simulink model "LM_TOS_0107_FIX"  (R2018b)
settings: Solver=FixedStepDiscrete  StartTime=0.0  StopTime=inf  FixedStep=0.005  RelTol=1e-3
PostLoadFcn:
  | if any(exist('dsrtsu_mdlpostloadfcn', 'file') ~= 0), dsrtsu_mdlpostloadfcn('Execute', bdroot); end
libraries: rtican x35
(part 1 of 11)
settings Model: DSRTSU_INTERNAL_RTI_VER=540  DSRTSU_INTERNAL_RTI_TYPE=rti1401  RTICANMMDATA=struct('GeneralSetupData',struct('modelroot','D:\00_Work\00_ZOP\00_ZOP_Demo_sim\LaneModel_20210107_1_CYX_FixHMI','generalsettings',struct('filesettings',struct('destfolder',struct('Name','RTICANMM_FILES','Check',1),'buildfolder',struct('Name','.','Check',1),'AbsDestfolder',struct('Name','D:\00_Work\00_ZOP\00_ZOP_Demo_sim\LaneModel_20210107_1_CYX_FixHMI\RTICANMM_FILES'),'AbsBuildfolder',struct('Name','D:\00_Work\00_ZOP\00_ZOP_Demo_sim\LaneModel_20210107_1_CYX_FixHMI'))),'options',struct('addpaths',1,'rmpaths',1,'addtrcexclusion',logical(1),'cannavigator',struct('checkmonitoring',0),'show_usrtrc',0,'use_usrtrc',0),'advanced',struct('options',ones(1,100)),'MPSetup',{{}},'RTI',struct('Type','RTI1401','Ver','7.12','Date','02-May-2019'),'modelname','LM_TOS','block','LM_TOS'))  DSRTSU_INTERNAL_RTIFPGA=130  Creator=only  LastModifiedBy=only
settings OptimizationCC: BlockReduction=off  ConditionallyExecuteInputs=off  DefaultUnderspecifiedDataType=single  BufferReuse=off  EnhancedBackFolding=on  ExpressionFolding=off  PassReuseOutputArgsThreshold=0  LocalBlockOutputs=off  OptimizeBlockOrder=speed  DifferentSizesBufferReuse=on
settings DebuggingCC: ParameterTunabilityLossMsg=error
settings HardwareCC: ProdBitPerPointer=32  ProdBitPerSizeT=32  ProdBitPerPtrDiffT=32  ProdLargestAtomicInteger=Integer  ProdEndianess=BigEndian  ProdWordSize=32  ProdHWDeviceType=Custom Processor->Custom  TargetIntDivRoundTo=Zero  TargetEndianess=BigEndian  TargetHWDeviceType=Custom Processor->Custom
settings ModelReferenceCC: ModelReferenceNumInstancesAllowed=Single
settings SFSimCC: MATLABDynamicMemAlloc=off
settings RTWCC: SystemTargetFile=rti1401.tlc  MakeCommand=make_rti  TemplateMakefile=rti1401.tmf  Description=dSPACE DS1401 Hardware Platform  GenerateReport=on  LaunchReport=on
settings CodeAppCC: OperatorAnnotations=on
settings STFCustomTargetCC: ParMdlRefBuildCompliant=on  SystemTargetFile=rti1401.tlc
settings GRTTargetCC: TargetLangStandard=C89/C90 (ANSI)  CompOptLevelCompliant=off  ConcurrentExecutionCompliant=off  CombineOutputUpdateFcns=off  MatFileLogging=off  CPPClassGenCompliant=off  UseToolchainInfoCompliant=off

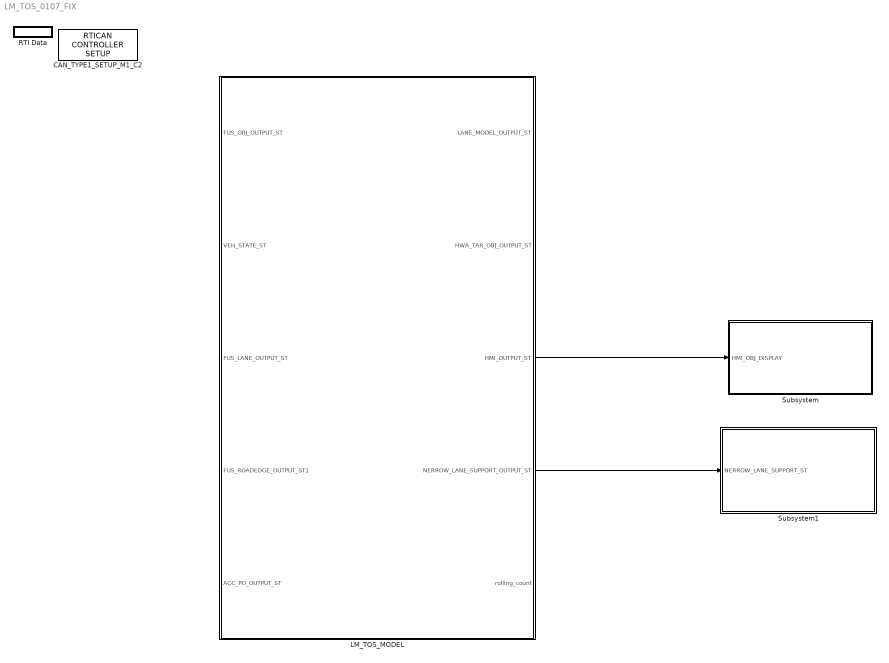
== system LM_TOS_0107_FIX ==
  CAN_TYPE1_SETUP_M1_C2 : rtican/RTICAN CONTROLLER SETUP   Reserved1=[]  Reserved2=[]  Reserved3=[]  Reserved4=[]  AcceptanceMask=[]  ArbitrationField=[]  Parameters=[]  SFcnRTICANSettings=[]  MS_Struct=[]  BoardTypeNo=[]  BoardNo=[]  ChannelNo=[]  DialogFcn=[]  UnitName=[]  Revision=[]  UnitValues=[]  DSProperties=struct('RTI',struct('Version',uint32(12),'BlockType',struct('isSLSource',uint8(0),'isSLSink',uint8(0),'isHWSource',uint8(0),'isHWSink',uint8(0),'isSetup',uint8(1),'isInline',uint8(1),'isNonInline',uint8(0),'isInterrupt',uint8(0),'isChannelwise',uint8(0)),'IOBoardType','RTICAN','UnitType','NON_MESSAGE','Identifier','MASTER','DialogType','ML','BlockSet','RTICAN','SlaveProcessor','CAN'))  RTIBlockInterface=struct('InputPortsWidth',int32(0),'InputPortsActive',0,'OutputPortsWidth',int32(0),'OutputPortsActive',0,'DialogFcn','rtican_master_setup_gui','BlockDisplay',{{['CAN CONTROLLER\n SETUP'],'center'}},'IconTransparency','on','InitLevel',3,'IWork',{{{'',uint32(2)}}},'BlockName',struct('Token',{{'CAN_TYPE','_SETUP_M','_C'}},'BlockParam',{{'BoardTypeNo','BoardNo','ChannelNo'}}),'ParameterTunableNames',{{}})  RTIBlockParameters="struct('BoardTypeNo',{{1,'OFF',[]}},'BoardNo',{{1,'ON',[1 16]}},'ChannelNo',{{2,'ON',[1 2]}},'AcceptanceMask',{{0,'OFF',[]}},'ArbitrationField',{{0,'OFF',[]}},'Parameters',{{struct('Config',struct('Baudrate',500,'SampleMode',1,'UsedParamSet',1,'validSettings',1,'isBTRvalues',0,'Advanced',struct('Baudrate',{500,500,500},'Frequency',{24000000,36000000,64000000},'Settings',{struct('SMPL',0,'BRP',0,'NBT',24,'TSEG1',15,'TSEG2',6,'SJW',3,'SP',70),struct('SMPL',0,'BRP',1,'NBT',18,'TSEG1',14,'TSEG2',1,'SJW',1,'SP',88),struct('SMPL',0,'BRP',3,'NBT',16,'TSEG1',12,'TSEG2',1,'SJW',1,'SP',87)},'BTR0',{192,65,67},'BTR1',{111,30,28})),'configType',1,'Options',struct('DataFileSelected',1,'DataFileName',{{'c:\\users\\only\\desktop\\mab_ipc_v1.8.dbc'}},'DataFileDate',{{['28-12月-2020 13:33:19']}},'InterfaceFcn','rtican_dbc_file_parser','InterfaceFcnFileName','','LabelConfigType','volatile','AcceptanceMaskSelected',0,'MsgDataType','AllwaysDouble','NumType','hex','MaskType','STD','AcceptanceMask',0,'ArbitrationField',0,'UseMultipleMessageAccess',0),'RxReceiveStdOptions',struct('RxServiceStdEnabled',0,'RxServiceStdMsgIdent',1000,'RxServiceStdIdentNumType',1,'RxServiceStdIdentMask',0,'RxServiceStdMaskNumType',1,'RxServiceStdQueueSize',64),'RxReceiveXtdOptions',struct('RxServiceXtdEnabled',0,'RxServiceXtdMsgIdent',1001,'RxServiceXtdIdentNumType',1,'RxServiceXtdIdentMask',0,'RxServiceXtdMaskNumType',1,'RxServiceXtdQueueSize',64),'PartialNetworkingOptions',struct('switchedon',0,'format',1,'idmask',['    XXXXX XXXXXXXX XXXXXXXX XXXXXXXX'],'idcode','0','idfilter','0','datamaskused',0,'datalength',1,'datamask','0x0000000000000000','partialnetworkenable',0),'general',struct('Termination_common',1,'Termination_C252',1,'BusConfigurationRegister',0,'Transceiver','ISO11898','isFromLib',0)),'OFF',[]}},'CCPParameters',{{struct('CRO',struct('Format','STD','NumFormat','hex','Id',1639),'DTO',struct('Format','STD','NumFormat','hex','Id',2017),'StationAdr',struct('NumFormat','hex','Value',57),'StationId',struct('Value',['dSPACE CCP Service']),'Enabled',0),'OFF',[]}},'XCPParameters',{{struct('MASTER',struct('Format','STD','NumFormat','hex','Id',256),'SLAVE',struct('Format','STD','NumFormat','hex','Id',510),'Enabled',0,'PIDTransmissionEnabled',0),'OFF',[]}},'GroupId',{{struct('Group',{{'RTICAN'}},'No',1,'Behavior',{{'EVER'}},'BlockType',{{'SOURCE'}},'NameChangeFlag',1),'OFF',[]}},'SFcnRTICANSettings',{{struct('Baudrate',500,'configType',1,'AdvancedConfig',struct('Frequency',{},'BTR0',{},'BTR1',{}),'UsedParamSet',1,'STDMaskSelected','no','XTDMaskSelected','no','BoardType','DS1','BoardNo',1,'ControllerNo',2,'Transceiver','ISO11898','BusConfigRegister',0,'TerminationRes',120,'UseMultipleMessageAccess','no','STDRXSrvcUsed','no','STDRXSrvcMsgId',1000,'STDRXSrvcMsgMask',0,'STDRXSrvcQueueSize',64,'XTDRXSrvcUsed','no','XTDRXSrvcMsgId',1001,'XTDRXSrvcQueueSize',64,'XTDRXSrvcMsgMask',0,'PN_IsPNTransciever',0,'PN_IsPNEnabled',0,'PN_MsgFormat',1,'PN_idcode',0,'PN_idmask',2047,'PN_datamaskused',0,'PN_datalength',0,'PN_datamask',['0xFF, 0xFF, 0xFF, 0xFF, 0xFF, 0xFF, 0xFF, 0xFF']),'OFF',[]}},'SFcnRTICCPSettings',{{struct('CRO',struct('Format','STD','NumFormat','hex','Id',1639),'DTO',struct('Format','STD','NumFormat','hex','Id',2017),'StationAdr',struct('NumFormat','hex','Value',57),'StationId',struct('Value',['dSPACE CCP Service']),'Enabled',0),'OFF',[]}},'SFcnRTIXCPSettings',{{struct('MASTER',struct('Format','STD','NumFormat','hex','Id',256),'SLAVE',struct('Format','STD','NumFormat','hex','Id',510),'Enabled',0,'PIDTransmissionEnabled',0),'OFF',[]}},'TLCFileName',{{'rtican_master_setup','OFF',[]}})"  RTISFcnParameters=struct('SFcnRTICANSettings','struct','SFcnRTICCPSettings','struct','SFcnRTIXCPSettings','struct','AcceptanceMask','int32','ArbitrationField','int32','TLCFileName','char')  RTIBlockParaDefault="struct('BoardTypeNo',4302,'BoardNo',1,'ChannelNo',1,'AcceptanceMask',0,'ArbitrationField',0,'Parameters',struct('Config',struct('Baudrate',500,'SampleMode',1,'UsedParamSet',1,'validSettings',1,'isBTRvalues',0,'Advanced',struct('Frequency',16000000,'BTR0',64,'BTR1',28,'Settings',struct('SMPL',0,'BRP',0,'NBT',16,'TSEG1',12,'TSEG2',1,'SJW',1,'SP',87))),'configType',1,'Options',struct('DataFileSelected',0,'DataFileName',{{['<no datafile support>']}},'DataFileDate',{{''}},'InterfaceFcn','rtican_dbc_file_parser','InterfaceFcnFileName','','LabelConfigType','volatile','AcceptanceMaskSelected',0,'MsgDataType','AllwaysDouble','NumType','hex','MaskType','STD','AcceptanceMask',0,'ArbitrationField',0,'UseMultipleMessageAccess',0),'RxReceiveStdOptions',struct('RxServiceStdEnabled',0,'RxServiceStdMsgIdent',1000,'RxServiceStdIdentNumType',1,'RxServiceStdIdentMask',0,'RxServiceStdMaskNumType',1,'RxServiceStdQueueSize',64),'RxReceiveXtdOptions',struct('RxServiceXtdEnabled',0,'RxServiceXtdMsgIdent',1001,'RxServiceXtdIdentNumType',1,'RxServiceXtdIdentMask',0,'RxServiceXtdMaskNumType',1,'RxServiceXtdQueueSize',64),'PartialNetworkingOptions',struct('switchedon',0,'format',1,'idmask',['    XXXXX XXXXXXXX XXXXXXXX XXXXXXXX'],'idcode','0','idfilter','0','datamaskused',0,'datalength',1,'datamask','0x0000000000000000','partialnetworkenable',0),'general',struct('Termination_common',1,'Termination_C252',1,'BusConfigurationRegister',0,'Transceiver','ISO11898','isFromLib',1)),'CCPParameters',struct('CRO',struct('Format','STD','NumFormat','hex','Id',1639),'DTO',struct('Format','STD','NumFormat','hex','Id',2017),'StationAdr',struct('NumFormat','hex','Value',57),'StationId',struct('Value',['dSPACE CCP Service']),'Enabled',0),'XCPParameters',struct('MASTER',struct('Format','STD','NumFormat','hex','Id',256),'SLAVE',struct('Format','STD','NumFormat','hex','Id',510),'Enabled',0,'PIDTransmissionEnabled',0),'GroupId',struct('Group',{{'RTICAN'}},'No',1,'Behavior',{{'EVER'}},'BlockType',{{'SOURCE'}},'NameChangeFlag',1),'SFcnRTICANSettings',struct('Baudrate',500,'configType',1,'AdvandedConfig',struct('Frequency',16000000,'BTR0','0x40','BTR1','0x1C'),'UsedParamSet',1,'STDMaskSelected','no','XTDMaskSelected','no','BoardType','DS4302','BoardNo',1,'ControllerNo',1,'Transceiver','ISO11898','BusConfigRegister',0,'TerminationRes',120,'UseMultipleMessageAccess','no','STDRXSrvcUsed','no','STDRXSrvcMsgId',1000,'STDRXSrvcMsgMask',0,'STDRXSrvcQueueSize',64,'XTDRXSrvcUsed','no','XTDRXSrvcMsgId',1001,'XTDRXSrvcQueueSize',64,'XTDRXSrvcMsgMask',0),'SFcnRTICCPSettings',struct('CRO',struct('Format','STD','NumFormat','hex','Id',1639),'DTO',struct('Format','STD','NumFormat','hex','Id',2017),'StationAdr',struct('NumFormat','hex','Value',57),'StationId',struct('Value',['dSPACE CCP Service']),'Enabled',0),'SFcnRTIXCPSettings',struct('MASTER',struct('Format','STD','NumFormat','hex','Id',256),'SLAVE',struct('Format','STD','NumFormat','hex','Id',510),'Enabled',0,'PIDTransmissionEnabled',0),'TLCFileName','rtican_master_setup')"
      settings: AttributesFormatString=Group Id: RTICAN1\n  SourceProductName=dSPACE RTI CAN Blockset
  LM_TOS_MODEL : Subsystem
  RTI Data : Subsystem  Tag=struct('RTIDataServer',struct('RTIDataServerVs','2','RTIModelDescription','struct(''main'',''LM_TOS'',''sub'','''',''isMp'',0)'))  LoadFcn="if exist('rtidc'), try,  rtidc('DataHostBlockClbLoad', gcbh); catch, disp(['Warning: ''LoadFcn'' for RTI Data block failed: ' lasterr]); end, end,"  mask(RTI_DATA_HOST){}
      mask help:
      | RTI Data Block.
      | This block is used by RTI to store internal model-dependent data.
      | Please keep this block on the root level of the model. Deleting this block will result in data loss.
      |
      | NEVER DELETE OR COPY THIS BLOCK!
      settings: CopyFcn="if exist('rtidc'), try,  rtidc('DataHostBlockClbCopy', gcbh); catch, disp(['Warning: ''CopyFcn'' for RTI Data block failed: ' lasterr]); end, end,"  DeleteFcn="if exist('rtidc'), try,  rtidc('DataHostBlockClbDelete', gcbh); catch, disp(['Warning: ''DeleteFcn'' for RTI Data block failed: ' lasterr]); end, end,"  ModelCloseFcn="if exist('rtidc'), try,  rtidc('DataHostBlockClbModelClose', gcbh); catch, disp(['Warning: ''ModelCloseFcn'' for RTI Data block failed: ' lasterr]); end, end,"  PreSaveFcn="if exist('rtidc'), try,  rtidc('DataHostBlockClbPreSave', gcbh); catch, disp(['Warning: ''PreSaveFcn'' for RTI Data block failed: ' lasterr]); end, end,"  PostSaveFcn="if exist('rtidc'), try,  rtidc('DataHostBlockClbPostSave', gcbh); catch, disp(['Warning: ''PostSaveFcn'' for RTI Data block failed: ' lasterr]); end, end,"  NameChangeFcn="if exist('rtidc'), try,  rtidc('DataHostBlockClbNameChange', gcbh); catch, disp(['Warning: ''NameChangeFcn'' for RTI Data block failed: ' lasterr]); end, end,"
      mask Help:
      | RTI Data Block.
      | This block is used by RTI to store internal model-dependent data.
      | Please keep this block on the root level of the model. Deleting this block will result in data loss.
      | 
      | NEVER DELETE OR COPY THIS BLOCK!
      mask Display:
      | text(0.5, 0.5, 'RTI Data', 'HorizontalAlignment', 'center');
      | plot([1 0]);
  Subsystem : Subsystem
  Subsystem1 : Subsystem
  wires:
  LM_TOS_MODEL/3(HMI_OUTPUT_ST) -> Subsystem/1(HMI_OBJ_DISPLAY)
  LM_TOS_MODEL/4(NERROW_LANE_SUPPORT_OUTPUT_ST) -> Subsystem1/1(NERROW_LANE_SUPPORT_ST)

== system LM_TOS_0107_FIX/LM_TOS_MODEL ==
  FUS_OBJ_OUTPUT_ST : Inport  OutDataTypeStr=Bus: FUS_OBJ_OUTPUT_ST
  VEH_STATE_ST : Inport  Port=2  OutDataTypeStr=Bus: VSI_VEHSTATE_ST
  FUS_LANE_OUTPUT_ST : Inport  Port=3  OutDataTypeStr=Bus: FUS_LANE_OUTPUT_ST
  FUS_ROADEDGE_OUTPUT_ST1 : Inport  Port=4  OutDataTypeStr=Bus: FUS_ROAD_EDGE_OUTPUT_ST
  ACC_PO_OUTPUT_ST : Inport  Port=5  OutDataTypeStr=Bus: ATS_PO_ST
  LM_TOS_ALGORISM : S-Function  InitFcn=try, set_param(gcb,'FunctionName','LM_TOS_MODULE'), end  FunctionName=LM_TOS_MODULE  SFunctionModules=LM_TOS_MODULE_wrapper Adapters LMBase LMMathLib LMPp LMTOSRunAlgo LMF TOSBase TOSHWA TOSPp VSL TOSNRA TOSTruckEvasion HMI CoordinationTransformation Parameters VehicleMovement DrivingManeuver LMCommonDefines  SFunctionDeploymentMode=off  EnableBusSupport=off  mask(S-Function Builder){}
      mask help: Simulink:masks:SFunctionBuilder_MD
      mask init:
      | val = [[.9  0.75 0.75 1 1 .9 .9 1]',[1 1 0.75 0.75 .9 .9 1 .9]'];try , sys = get_param(gcb,'SfunBuilderFcnName');if isempty(sys), sys = get_param(gcb,'FunctionName'); end,catch, sys = get_param(gcb,'FunctionName'); end
      settings: CopyFcn=set_param(gcbh,'LinkStatus','none')  PreSaveFcn=try, set_param(gcb,'FunctionName','LM_TOS_MODULE'), end  OpenFcn=sfunctionwizard(gcbh)
      mask Display:
      | plot(val(:,1),val(:,2))
      | disp(sys)
      | port_label('input',1,'timeStamp_In')
      | port_label('input',2,'frameNum_In')
      | port_label('input',3,'objects_In')
      | port_label('input',4,'vehState_In')
      | port_label('input',5,'fus_Lane_In')
      | port_label('input',6,'fus_roadEdge_In')
      | port_label('input',7,'acc_to_In')
      | port_label('output',1,'egoLaneId_output')
      | port_label('output',2,'lanes_bas_info_st_output')
      | port_label('output',3,'tar_obj_st_output')
      | port_label('output',4,'segments_st_output')
      | port_label('output',5,'hwa_tar_obj_st_output')
      | port_label('output',6,'hmi_obj_count_output')
      | port_label('output',7,'hmi_info_st_output')
      | port_label('output',8,'nls_info_st_output')
      | port_label('output',9,'rolling_count_output')
  adapter1 : Subsystem
  adapter2 : Subsystem
  LANE_MODEL_OUTPUT_ST : Outport  OutDataTypeStr=Bus: LANEMODEL_OUTPUT_ST
  HWA_TAR_OBJ_OUTPUT_ST : Outport  Port=2  OutDataTypeStr=Bus: HWA_TARGETOBJECT_OUTPUT_ST
  HMI_OUTPUT_ST : Outport  Port=3  OutDataTypeStr=Bus: HMI_OUTPUT_ST
  NERROW_LANE_SUPPORT_OUTPUT_ST : Outport  Port=4  OutDataTypeStr=Bus: NARROW_LANE_SUPPORT_OUTPUT_ST
  rolling_count : Outport  Port=5  OutDataTypeStr=uint16
  wires:
  LM_TOS_ALGORISM/4 -> adapter2/4(segments_st_adp)
  VEH_STATE_ST/1 -> adapter1/2(Veh_State_st)
  adapter1/1(timeStamp) -> LM_TOS_ALGORISM/1
  LM_TOS_ALGORISM/2 -> adapter2/2(LANES_BAS_INFO_ST_adp)
  adapter1/3(objects) -> LM_TOS_ALGORISM/3
  LM_TOS_ALGORISM/3 -> adapter2/3(tar_objs_st_adp)
  adapter1/5(fus_lane_output) -> LM_TOS_ALGORISM/5
  FUS_OBJ_OUTPUT_ST/1 -> adapter1/1(Fus_obj_outPut_st)
  adapter1/2(frameNum) -> LM_TOS_ALGORISM/2
  LM_TOS_ALGORISM/5 -> adapter2/5(hwa_tar_obj_output_st)
  adapter1/4(veh_state) -> LM_TOS_ALGORISM/4
  LM_TOS_ALGORISM/1 -> adapter2/1(egoLaneId)
  adapter2/2(hwa_target_object_output_st) -> HWA_TAR_OBJ_OUTPUT_ST/1
  adapter2/1(Lane_model_output_st) -> LANE_MODEL_OUTPUT_ST/1
  FUS_LANE_OUTPUT_ST/1 -> adapter1/3(Fus_Lane_output_st)
  FUS_ROADEDGE_OUTPUT_ST1/1 -> adapter1/4(Fus_RoadEdge_output_st)
  adapter1/6(fus_RoadEdge_output) -> LM_TOS_ALGORISM/6
  adapter2/3(hmi_display_info_st) -> HMI_OUTPUT_ST/1
  LM_TOS_ALGORISM/6 -> adapter2/6(hmi_display_obj_count)
  LM_TOS_ALGORISM/7 -> adapter2/7(hmi_display_st_apt)
  LM_TOS_ALGORISM/8 -> adapter2/8(hmi_display_st_apt1)
  ACC_PO_OUTPUT_ST/1 -> adapter1/5(acc_po_output_st)
  adapter1/7(acc_po_st) -> LM_TOS_ALGORISM/7
  adapter2/4(nls_info_st) -> NERROW_LANE_SUPPORT_OUTPUT_ST/1
  LM_TOS_ALGORISM/9 -> rolling_count/1

== system LM_TOS_0107_FIX/RTI Data ==
  RTI Data Store : Subsystem  Tag="struct('private',struct('version',struct('dsVer',uint32(2),'dsVerCreation',uint32(2),'RTI',struct('ver','7.12','type','RTI1401')),'access',struct('type','Model','isPerm',1,'created',['30-Dec-2020 15:54:56'],'modified',['15-Jan-2021 08:25:17'],'location','')),'public',struct('main',struct('data',[]),'sub',struct('name',{{'LM_TOS'}},'data',{{struct('TH',struct('thTaskInfo',struct('taskType',{'TIMER','HWINT','TMRINT','SWINT','GLINT'},'tasksNumOf',{1,0,0,0,0},'srcIds',{{'TIMERA'},{},{},{},{}},'taskNames',{{['Timer Task 1']},{},{},{},{}})),'th_tc',struct('dataType','TASK','taskGroupId','','taskGroupList',{{}},'taskSchedulingPolicy','FCFS','taskType','TIMER','blkh',-1,'srcId','TIMERA','srcSgnName',['Timer A interrupt'],'srcCpuName','','taskName',['Timer Task 1  [0.005] s'],'taskNameDisplayExt','','smplTime',0.005,'smplTimeOffs',0,'hasFixedPriority',0,'priority',1,'hasFixedOvc',0,'ovcType',1,'ovcMax',1),'tc_th',struct('dataType','TASK','taskGroupId','','taskGroupList',{{}},'taskSchedulingPolicy','FCFS','taskType','TIMER','blkh',-1,'srcId','TIMERA','srcSgnName',['Timer A interrupt'],'srcCpuName','','taskName',['Timer Task 1  [0.005] s'],'taskNameDisplayExt','','smplTime',0.005,'smplTimeOffs',0,'hasFixedPriority',0,'priority',1,'hasFixedOvc',0,'ovcType',1,'ovcMax',1))}})))"  mask(RTI_DATA_STORE){}
      mask help:
      | RTI Data Store Block. This block is used by RTI to store internal model dependent data. Deleting this block will result in data loss.
      |
      | NEVER DELETE, COPY, OR MODIFY THIS BLOCK!
      mask Help:
      | RTI Data Store Block. This block is used by RTI to store internal model dependent data. Deleting this block will result in data loss.
      | 
      | NEVER DELETE, COPY, OR MODIFY THIS BLOCK!
      mask Display: text(0.5, 0.5, ' ', 'HorizontalAlignment', 'center');

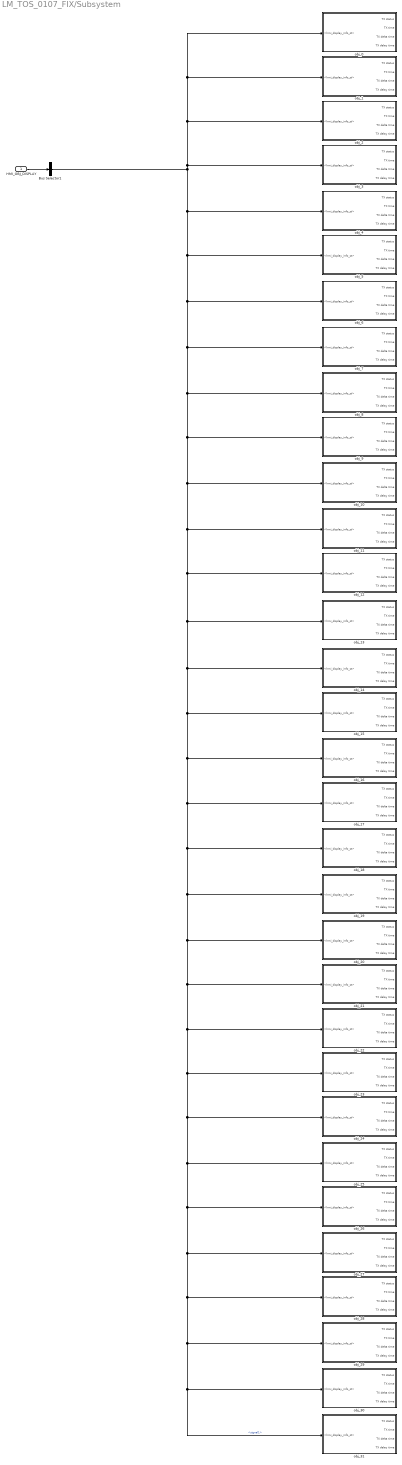
== system LM_TOS_0107_FIX/Subsystem ==
  HMI_OBJ_DISPLAY : Inport  OutDataTypeStr=Bus: HMI_OUTPUT_ST
  Bus Selector1 : BusSelector  OutputSignals=signal2.signal1
  obj_0 : Subsystem
  obj_1 : Subsystem
  obj_10 : Subsystem
  obj_11 : Subsystem
  obj_12 : Subsystem
  obj_13 : Subsystem
  obj_14 : Subsystem
  obj_15 : Subsystem
  obj_16 : Subsystem
  obj_17 : Subsystem
  obj_18 : Subsystem
  obj_19 : Subsystem
  obj_2 : Subsystem
  obj_20 : Subsystem
  obj_21 : Subsystem
  obj_22 : Subsystem
  obj_23 : Subsystem
  obj_24 : Subsystem
  obj_25 : Subsystem
  obj_26 : Subsystem
  obj_27 : Subsystem
  obj_28 : Subsystem
  obj_29 : Subsystem
  obj_3 : Subsystem
  obj_30 : Subsystem
  obj_31 : Subsystem
  obj_4 : Subsystem
  obj_5 : Subsystem
  obj_6 : Subsystem
  obj_7 : Subsystem
  obj_8 : Subsystem
  obj_9 : Subsystem
  wires:
  HMI_OBJ_DISPLAY/1 -> Bus Selector1/1
  Bus Selector1/1 -> obj_3/1(<hmi_display_info_st>), obj_2/1(<hmi_display_info_st>), obj_1/1(<hmi_display_info_st>), obj_0/1(<hmi_display_info_st>), obj_4/1(<hmi_display_info_st>), obj_5/1(<hmi_display_info_st>), obj_6/1(<hmi_display_info_st>), obj_7/1(<hmi_display_info_st>), obj_9/1(<hmi_display_info_st>), obj_10/1(<hmi_display_info_st>), obj_11/1(<hmi_display_info_st>), obj_12/1(<hmi_display_info_st>), obj_13/1(<hmi_display_info_st>), obj_14/1(<hmi_display_info_st>), obj_15/1(<hmi_display_info_st>), obj_16/1(<hmi_display_info_st>), obj_17/1(<hmi_display_info_st>), obj_18/1(<hmi_display_info_st>), obj_19/1(<hmi_display_info_st>), obj_20/1(<hmi_display_info_st>), obj_21/1(<hmi_display_info_st>), obj_22/1(<hmi_display_info_st>), obj_23/1(<hmi_display_info_st>), obj_24/1(<hmi_display_info_st>), obj_27/1(<hmi_display_info_st>), obj_28/1(<hmi_display_info_st>), obj_29/1(<hmi_display_info_st>), obj_30/1(<hmi_display_info_st>), obj_31/1(<hmi_display_info_st>), obj_26/1(<hmi_display_info_st>), obj_25/1(<hmi_display_info_st>), obj_8/1(<hmi_display_info_st>)  "<signal1>"

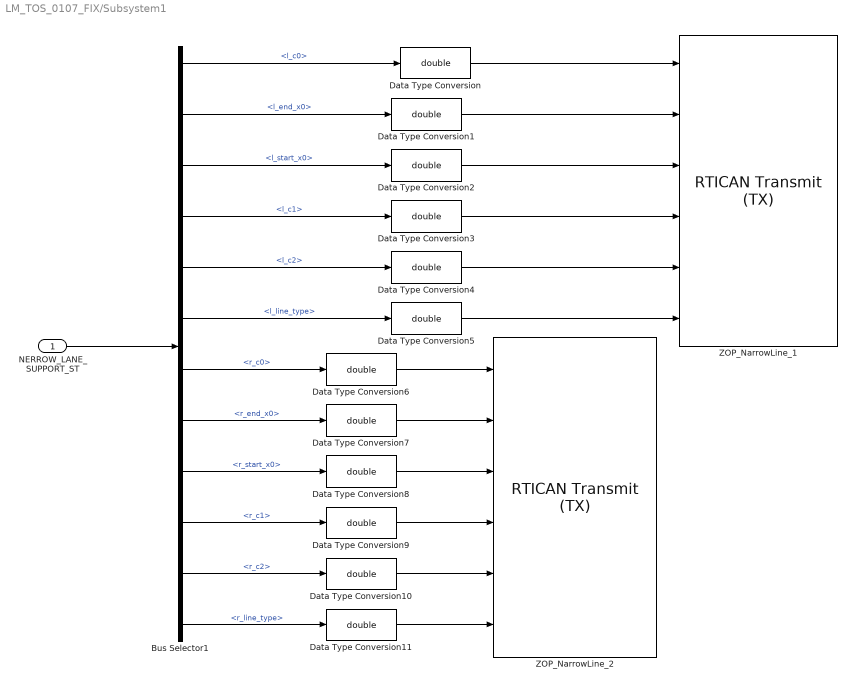
== system LM_TOS_0107_FIX/Subsystem1 ==
  NERROW_LANE_SUPPORT_ST : Inport  OutDataTypeStr=Bus: NARROW_LANE_SUPPORT_OUTPUT_ST
  Bus Selector1 : BusSelector  OutputSignals=l_c0,l_end_x0,l_start_x0,l_c1,l_c2,l_line_type,r_c0,r_end_x0,r_start_x0,r_c1,r_c2,r_line_type
  Data Type Conversion{,1..11} (12 alike) : DataTypeConversion  OutDataTypeStr=double
  ZOP_NarrowLine_1 : rtican/RTICAN Transmit (TX)   Reserved1=[]  Reserved2=[]  Reserved3=[]  Reserved4=[]  SfcnMessage=[]  Msg_Struct=[]  BoardTypeNo=[]  BoardNo=[]  ChannelNo=[]  Parameters=[]  DialogFcn=[]  UnitName=[]  Revision=[]  UnitValues=[]  DSProperties=struct('RTI',struct('Version',uint32(5),'BlockType',struct('isSLSource',uint8(1),'isSLSink',uint8(1),'isHWSource',uint8(0),'isHWSink',uint8(0),'isSetup',uint8(0),'isInline',uint8(1),'isNonInline',uint8(0),'isInterrupt',uint8(0),'isChannelwise',uint8(0)),'IOBoardType','RTICAN','UnitType','MESSAGE','Identifier','TX','DialogType','MSVC','BlockSet','RTICAN','SlaveProcessor','CAN'))  RTIBlockInterface=struct('InputPortsWidth',int32([1 1 1 1 1 1]),'InputPortsActive',[1 1 1 1 1 1],'InputPortsName',{{'Lane_C0','ZOP_narrowLane_dxEnd','ZOP_narrowLane_dxStart','Lane_C1','Lane_C2','ZOP_narrowLaneType'}},'InputPortsDataType',{{'SS_DOUBLE','SS_DOUBLE','SS_DOUBLE','SS_DOUBLE','SS_DOUBLE','SS_DOUBLE'}},'OutputPortsWidth',int32([1 1 1 1]),'OutputPortsActive',[1 1 1 1],'OutputPortsName',{{['TX status'],['TX time'],['TX delta time'],['TX delay time']}},'DialogFcn','rtican_message_interface_gui','BlockDisplay',{{'','center'}},'IconTransparency','on','InitLevel',3,'BlockName',struct('Token',{{'ZOP_NarrowLine_1'}}),'SampleTime',{{-1}},'TriggerPort',{{'none'}},'EnablePort',{{'none'}})  RTIBlockParameters=struct('BoardTypeNo',{{1,'OFF',[]}},'BoardNo',{{1,'ON',[1 16]}},'ChannelNo',{{2,'ON',[1 2]}},'Parameters',{{struct('DataFileSupport',struct('DataFileSelectedMaster',1,'DataFileSelectedLocal',1,'DataFileName','c:\users\only\desktop\mab_ipc_v1.8.dbc|','DataFileDate',{{{['28-12月-2020 13:33:19']}}},'SelectedFile','c:\users\only\desktop\mab_ipc_v1.8.dbc'),'Options',struct('StatusSelected',1,'TimeSelected',1,'DeltaTimeSelected',1,'DelayTimeSelected',1,'DelayTimeTXCommandSelected',0,'EncodeSetUnusedBitsToOne',0,'EnableMsgLoopback',0,'TriggerPort',struct('Selected',0,'TriggerType',0),'EnablePortSelected',0,'SignalOnPortnameSelected',1,'UserCoding',struct('Selected',0,'InterfaceFile','UserEncodingFile','FcnName','UserEncodeFcn','InportSelected',0,'InportWidth',1,'OutportSelected',0,'OutportWidth',1),'TerminationMsg',struct('Selected',0,'Byte0_7','0'),'InitialMsg',struct('Selected',0,'Byte0_7','0')),'Message',struct('MsgOnBlocknameSelected',1,'MsgName','ZOP_NarrowLine_1','MsgIdFormat',0,'MsgId',570,'MsgLength',8,'NumSignals',6,'SampleTime',-1,'StartTime',struct('Selected',0,'Value',0),'AutoRepeatTime',struct('Selected',0,'Value',0.1),'Timeout',struct('Selected',0,'Value',0.1),'DelayTime',struct('Selected',0,'Value',0.1),'Signal',struct('SgnName',{'Lane_C0','ZOP_narrowLane_dxEnd','ZOP_narrowLane_dxStart','Lane_C1','Lane_C2','ZOP_narrowLaneType'},'SgnStartBit',{0,0,12,16,28,52},'SgnLength',{12,12,12,11,12,4},'SgnType',{0,0,0,0,0,0},'ModeValue',{-1,-1,-1,-1,-1,-1},'DataType',{0,0,0,0,0,0},'ByteLayout',{0,2,2,0,0,2},'Factor',{0.01,0.01,0.01,0.0009,5e-6,1},'Offset',{-16,0,0,-0.9,-0.01,0},'SgnComment',{{['' char(10) '']},{''},{''},{''},{''},{''}},'SgnUnit',{'M','','','','',''},'Min',{-16,0,0,-0.9,-0.01,0},'Max',{15.99,40.95,40.95,0.9,0.01,15},'SLDataType',{'SS_DOUBLE','SS_DOUBLE','SS_DOUBLE','SS_DOUBLE','SS_DOUBLE','SS_DOUBLE'}),'MsgIdNumFormat',0,'MsgComment',{{''}}),'Version',1.2,'general',struct('isFromLib',0)),'OFF',[]}},'GroupId',{{struct('Group',{{'RTICAN'}},'No',1,'Behavior',{{'NAMECHANGE'}},'BlockType',{{'SINK'}},'NameChangeFlag',0),'OFF',[]}},'SFcnRTICANMessage',{{struct('MsgType','TX','SFcnPortType','Scalar','MsgName','ZOP_NarrowLine_1','MsgIdFormat','STD','MsgId',570,'MsgLength',8,'NumSignals',6,'SampleTime',-1,'StartTime',struct('Selected','no','Value',0),'AutoRepeatTime',struct('Selected','no','Value',0.1),'Timeout',struct('Selected','no','Value',0.1),'Signal',struct('SgnName',{'Lane_C0','ZOP_narrowLane_dxEnd','ZOP_narrowLane_dxStart','Lane_C1','Lane_C2','ZOP_narrowLaneType'},'SgnStartBit',{0,0,12,16,28,52},'SgnLength',{12,12,12,11,12,4},'SgnType',{'standard','standard','standard','standard','standard','standard'},'ModeValue',{-1,-1,-1,-1,-1,-1},'DataType',{['unsigned int'],['unsigned int'],['unsigned int'],['unsigned int'],['unsigned int'],['unsigned int']},'ByteLayout',{['little endian'],['motorola back.'],['motorola back.'],['little endian'],['little endian'],['motorola back.']},'Factor',{0.01,0.01,0.01,0.0009,5e-6,1},'Offset',{-16,0,0,-0.9,-0.01,0},'SLDataType',{'SS_DOUBLE','SS_DOUBLE','SS_DOUBLE','SS_DOUBLE','SS_DOUBLE','SS_DOUBLE'}),'StatusSelected','yes','TimeSelected','yes','DeltaTimeSelected','yes','DelayTimeSelected','yes','DelayTimeTXCommandSelected','no','EncodeSetUnusedBitsToOne','no','EnableMsgLoopback','no','TriggerPort',struct('Selected','no','TriggerType',0),'EnablePortSelected','no','UserCoding',struct('Selected','no','InterfaceFile','UserEncodingFile','FcnName','UserEncodeFcn','InportSelected','no','InportWidth',1,'OutportSelected','no','OutportWidth',1),'TerminationMsg',struct('Selected','no','Byte0','0x00','Byte1','0x00','Byte2','0x00','Byte3','0x00','Byte4','0x00','Byte5','0x00','Byte6','0x00','Byte7','0x00'),'InitialMsg',struct('Selected','no','Byte0','0x00','Byte1','0x00','Byte2','0x00','Byte3','0x00','Byte4','0x00','Byte5','0x00','Byte6','0x00','Byte7','0x00'),'BoardType','DS1','BoardNo',1,'ControllerNo',2),'OFF',[]}},'TLCFileName',{{'rtican_tx_message','OFF',[]}})  RTISFcnParameters=struct('SFcnRTICANMessage','struct','TLCFileName','char')  RTIBlockParaDefault=struct('BoardTypeNo',4302,'BoardNo',1,'ChannelNo',1,'Parameters',struct('DataFileSupport',struct('DataFileSelectedMaster',0,'DataFileSelectedLocal',0,'DataFileName','','DataFileDate','','SelectedFile',['<no file selected>']),'Options',struct('StatusSelected',1,'TimeSelected',1,'DeltaTimeSelected',1,'DelayTimeSelected',1,'DelayTimeTXCommandSelected',0,'EncodeSetUnusedBitsToOne',0,'EnableMsgLoopback',0,'TriggerPort',struct('Selected',0,'TriggerType','rising'),'EnablePortSelected',0,'SignalOnPortnameSelected',1,'UserCoding',struct('Selected',0,'InterfaceFile','UserEncodingFile','FcnName','UserEncodeFcn','InportSelected',0,'InportWidth',1,'OutportSelected',0,'OutportWidth',1),'TerminationMsg',struct('Selected',0,'Byte0_7','0'),'InitialMsg',struct('Selected',0,'Byte0_7','0')),'Message',struct('MsgOnBlocknameSelected',0,'MsgName',['TX Message'],'MsgIdFormat',0,'MsgId',100,'MsgLength',8,'NumSignals',1,'SampleTime',-1,'StartTime',struct('Selected',0,'Value',0),'AutoRepeatTime',struct('Selected',0,'Value',0.1),'Timeout',struct('Selected',0,'Value',0.1),'DelayTime',struct('Selected',0,'Value',0.1),'Signal',struct('SgnName',['TX signal'],'SgnStartBit',0,'SgnLength',8,'SgnType',0,'ModeValue',-1,'DataType',0,'SLDataType','SS_DOUBLE','ByteLayout',0,'Factor',1,'Offset',0,'Min',0,'Max',255,'SgnComment',{{}},'SgnUnit',''),'MsgIdNumFormat',0,'MsgComment',{{''}}),'Version',1.2,'general',struct('isFromLib',1)),'GroupId',struct('Group',{{'RTICAN'}},'No',1,'Behavior',{{'NAMECHANGE'}},'BlockType',{{'SINK'}},'NameChangeFlag',0),'SFcnRTICANMessage',struct('MsgType','TX','MsgName',['TX Message'],'MsgIdFormat','STD','MsgId',100,'MsgLength',2,'NumSignals',1,'SampleTime',-1,'StartTime',struct('Selected','no','Value',0),'AutoRepeatTime',struct('Selected','no','Value',0.1),'Timeout',struct('Selected','no','Value',0.1),'DelayTime',struct('Selected','no','Value',0.1),'Signal',struct('SgnName',['TX signal'],'SgnStartBit',0,'SgnLength',8,'SgnType','standard','ModeValue',-1,'DataType',['unsigned int'],'ByteLayout',['little endian'],'SLDataType','SS_DOUBLE','Factor',1,'Offset',0),'StatusSelected','yes','TimeSelected','yes','DeltaTimeSelected','yes','DelayTimeSelected','yes','EnablePortSelected','no','EnableMsgLoopback','no','DelayTimeTXCommandSelected','no','EncodeSetUnusedBitsToOne','no','UserCoding',struct('Selected','no','InterfaceFile','UserDecodingFile','FcnName','UserDecodeFcn','InportSelected','no','InportWidth',1,'OutportSelected','no','OutportWidth',1),'TerminationMsg',struct('Selected','no','Byte0','0x00','Byte1','0x00','Byte2','0x00','Byte3','0x00','Byte4','0x00','Byte5','0x00','Byte6','0x00','Byte7','0x00'),'InitialMsg',struct('Selected','no','Byte0','0x00','Byte1','0x00','Byte2','0x00','Byte3','0x00','Byte4','0x00','Byte5','0x00','Byte6','0x00','Byte7','0x00'),'TriggerPort',struct('Selected','no','TriggerType','rising'),'BoardType','DS4302','BoardNo',1,'ControllerNo',1,'SFcnPortType','Scalar'),'TLCFileName','rtican_tx_message')
      settings: AttributesFormatString=Group Id: RTICAN1\n  SourceProductName=dSPACE RTI CAN Blockset
  ZOP_NarrowLine_2 : rtican/RTICAN Transmit (TX)   Reserved1=[]  Reserved2=[]  Reserved3=[]  Reserved4=[]  SfcnMessage=[]  Msg_Struct=[]  BoardTypeNo=[]  BoardNo=[]  ChannelNo=[]  Parameters=[]  DialogFcn=[]  UnitName=[]  Revision=[]  UnitValues=[]  DSProperties=struct('RTI',struct('Version',uint32(5),'BlockType',struct('isSLSource',uint8(1),'isSLSink',uint8(1),'isHWSource',uint8(0),'isHWSink',uint8(0),'isSetup',uint8(0),'isInline',uint8(1),'isNonInline',uint8(0),'isInterrupt',uint8(0),'isChannelwise',uint8(0)),'IOBoardType','RTICAN','UnitType','MESSAGE','Identifier','TX','DialogType','MSVC','BlockSet','RTICAN','SlaveProcessor','CAN'))  RTIBlockInterface=struct('InputPortsWidth',int32([1 1 1 1 1 1]),'InputPortsActive',[1 1 1 1 1 1],'InputPortsName',{{'Lane_C0','ZOP_narrowLane_dxEnd','ZOP_narrowLane_dxStart','Lane_C1','Lane_C2','ZOP_narrowLaneType'}},'InputPortsDataType',{{'SS_DOUBLE','SS_DOUBLE','SS_DOUBLE','SS_DOUBLE','SS_DOUBLE','SS_DOUBLE'}},'OutputPortsWidth',int32([1 1 1 1]),'OutputPortsActive',[1 1 1 1],'OutputPortsName',{{['TX status'],['TX time'],['TX delta time'],['TX delay time']}},'DialogFcn','rtican_message_interface_gui','BlockDisplay',{{'','center'}},'IconTransparency','on','InitLevel',3,'BlockName',struct('Token',{{'ZOP_NarrowLine_2'}}),'SampleTime',{{-1}},'TriggerPort',{{'none'}},'EnablePort',{{'none'}})  RTIBlockParameters=struct('BoardTypeNo',{{1,'OFF',[]}},'BoardNo',{{1,'ON',[1 16]}},'ChannelNo',{{2,'ON',[1 2]}},'Parameters',{{struct('DataFileSupport',struct('DataFileSelectedMaster',1,'DataFileSelectedLocal',1,'DataFileName','c:\users\only\desktop\mab_ipc_v1.8.dbc|','DataFileDate',{{{['28-12月-2020 13:33:19']}}},'SelectedFile','c:\users\only\desktop\mab_ipc_v1.8.dbc'),'Options',struct('StatusSelected',1,'TimeSelected',1,'DeltaTimeSelected',1,'DelayTimeSelected',1,'DelayTimeTXCommandSelected',0,'EncodeSetUnusedBitsToOne',0,'EnableMsgLoopback',0,'TriggerPort',struct('Selected',0,'TriggerType',0),'EnablePortSelected',0,'SignalOnPortnameSelected',1,'UserCoding',struct('Selected',0,'InterfaceFile','UserEncodingFile','FcnName','UserEncodeFcn','InportSelected',0,'InportWidth',1,'OutportSelected',0,'OutportWidth',1),'TerminationMsg',struct('Selected',0,'Byte0_7','0'),'InitialMsg',struct('Selected',0,'Byte0_7','0')),'Message',struct('MsgOnBlocknameSelected',1,'MsgName','ZOP_NarrowLine_2','MsgIdFormat',0,'MsgId',571,'MsgLength',8,'NumSignals',6,'SampleTime',-1,'StartTime',struct('Selected',0,'Value',0),'AutoRepeatTime',struct('Selected',0,'Value',0.1),'Timeout',struct('Selected',0,'Value',0.1),'DelayTime',struct('Selected',0,'Value',0.1),'Signal',struct('SgnName',{'Lane_C0','ZOP_narrowLane_dxEnd','ZOP_narrowLane_dxStart','Lane_C1','Lane_C2','ZOP_narrowLaneType'},'SgnStartBit',{0,0,12,16,28,52},'SgnLength',{12,12,12,11,12,4},'SgnType',{0,0,0,0,0,0},'ModeValue',{-1,-1,-1,-1,-1,-1},'DataType',{0,0,0,0,0,0},'ByteLayout',{0,2,2,0,0,2},'Factor',{0.01,0.01,0.01,0.0009,5e-6,1},'Offset',{-16,0,0,-0.9,-0.01,0},'SgnComment',{{['' char(10) '']},{''},{''},{''},{''},{''}},'SgnUnit',{'M','','','','',''},'Min',{-16,0,0,-0.9,-0.01,0},'Max',{15.99,40.95,40.95,0.9,0.01,15},'SLDataType',{'SS_DOUBLE','SS_DOUBLE','SS_DOUBLE','SS_DOUBLE','SS_DOUBLE','SS_DOUBLE'}),'MsgIdNumFormat',0,'MsgComment',{{''}}),'Version',1.2,'general',struct('isFromLib',0)),'OFF',[]}},'GroupId',{{struct('Group',{{'RTICAN'}},'No',1,'Behavior',{{'NAMECHANGE'}},'BlockType',{{'SINK'}},'NameChangeFlag',0),'OFF',[]}},'SFcnRTICANMessage',{{struct('MsgType','TX','SFcnPortType','Scalar','MsgName','ZOP_NarrowLine_2','MsgIdFormat','STD','MsgId',571,'MsgLength',8,'NumSignals',6,'SampleTime',-1,'StartTime',struct('Selected','no','Value',0),'AutoRepeatTime',struct('Selected','no','Value',0.1),'Timeout',struct('Selected','no','Value',0.1),'Signal',struct('SgnName',{'Lane_C0','ZOP_narrowLane_dxEnd','ZOP_narrowLane_dxStart','Lane_C1','Lane_C2','ZOP_narrowLaneType'},'SgnStartBit',{0,0,12,16,28,52},'SgnLength',{12,12,12,11,12,4},'SgnType',{'standard','standard','standard','standard','standard','standard'},'ModeValue',{-1,-1,-1,-1,-1,-1},'DataType',{['unsigned int'],['unsigned int'],['unsigned int'],['unsigned int'],['unsigned int'],['unsigned int']},'ByteLayout',{['little endian'],['motorola back.'],['motorola back.'],['little endian'],['little endian'],['motorola back.']},'Factor',{0.01,0.01,0.01,0.0009,5e-6,1},'Offset',{-16,0,0,-0.9,-0.01,0},'SLDataType',{'SS_DOUBLE','SS_DOUBLE','SS_DOUBLE','SS_DOUBLE','SS_DOUBLE','SS_DOUBLE'}),'StatusSelected','yes','TimeSelected','yes','DeltaTimeSelected','yes','DelayTimeSelected','yes','DelayTimeTXCommandSelected','no','EncodeSetUnusedBitsToOne','no','EnableMsgLoopback','no','TriggerPort',struct('Selected','no','TriggerType',0),'EnablePortSelected','no','UserCoding',struct('Selected','no','InterfaceFile','UserEncodingFile','FcnName','UserEncodeFcn','InportSelected','no','InportWidth',1,'OutportSelected','no','OutportWidth',1),'TerminationMsg',struct('Selected','no','Byte0','0x00','Byte1','0x00','Byte2','0x00','Byte3','0x00','Byte4','0x00','Byte5','0x00','Byte6','0x00','Byte7','0x00'),'InitialMsg',struct('Selected','no','Byte0','0x00','Byte1','0x00','Byte2','0x00','Byte3','0x00','Byte4','0x00','Byte5','0x00','Byte6','0x00','Byte7','0x00'),'BoardType','DS1','BoardNo',1,'ControllerNo',2),'OFF',[]}},'TLCFileName',{{'rtican_tx_message','OFF',[]}})  RTISFcnParameters=struct('SFcnRTICANMessage','struct','TLCFileName','char')  RTIBlockParaDefault=struct('BoardTypeNo',4302,'BoardNo',1,'ChannelNo',1,'Parameters',struct('DataFileSupport',struct('DataFileSelectedMaster',0,'DataFileSelectedLocal',0,'DataFileName','','DataFileDate','','SelectedFile',['<no file selected>']),'Options',struct('StatusSelected',1,'TimeSelected',1,'DeltaTimeSelected',1,'DelayTimeSelected',1,'DelayTimeTXCommandSelected',0,'EncodeSetUnusedBitsToOne',0,'EnableMsgLoopback',0,'TriggerPort',struct('Selected',0,'TriggerType','rising'),'EnablePortSelected',0,'SignalOnPortnameSelected',1,'UserCoding',struct('Selected',0,'InterfaceFile','UserEncodingFile','FcnName','UserEncodeFcn','InportSelected',0,'InportWidth',1,'OutportSelected',0,'OutportWidth',1),'TerminationMsg',struct('Selected',0,'Byte0_7','0'),'InitialMsg',struct('Selected',0,'Byte0_7','0')),'Message',struct('MsgOnBlocknameSelected',0,'MsgName',['TX Message'],'MsgIdFormat',0,'MsgId',100,'MsgLength',8,'NumSignals',1,'SampleTime',-1,'StartTime',struct('Selected',0,'Value',0),'AutoRepeatTime',struct('Selected',0,'Value',0.1),'Timeout',struct('Selected',0,'Value',0.1),'DelayTime',struct('Selected',0,'Value',0.1),'Signal',struct('SgnName',['TX signal'],'SgnStartBit',0,'SgnLength',8,'SgnType',0,'ModeValue',-1,'DataType',0,'SLDataType','SS_DOUBLE','ByteLayout',0,'Factor',1,'Offset',0,'Min',0,'Max',255,'SgnComment',{{}},'SgnUnit',''),'MsgIdNumFormat',0,'MsgComment',{{''}}),'Version',1.2,'general',struct('isFromLib',1)),'GroupId',struct('Group',{{'RTICAN'}},'No',1,'Behavior',{{'NAMECHANGE'}},'BlockType',{{'SINK'}},'NameChangeFlag',0),'SFcnRTICANMessage',struct('MsgType','TX','MsgName',['TX Message'],'MsgIdFormat','STD','MsgId',100,'MsgLength',2,'NumSignals',1,'SampleTime',-1,'StartTime',struct('Selected','no','Value',0),'AutoRepeatTime',struct('Selected','no','Value',0.1),'Timeout',struct('Selected','no','Value',0.1),'DelayTime',struct('Selected','no','Value',0.1),'Signal',struct('SgnName',['TX signal'],'SgnStartBit',0,'SgnLength',8,'SgnType','standard','ModeValue',-1,'DataType',['unsigned int'],'ByteLayout',['little endian'],'SLDataType','SS_DOUBLE','Factor',1,'Offset',0),'StatusSelected','yes','TimeSelected','yes','DeltaTimeSelected','yes','DelayTimeSelected','yes','EnablePortSelected','no','EnableMsgLoopback','no','DelayTimeTXCommandSelected','no','EncodeSetUnusedBitsToOne','no','UserCoding',struct('Selected','no','InterfaceFile','UserDecodingFile','FcnName','UserDecodeFcn','InportSelected','no','InportWidth',1,'OutportSelected','no','OutportWidth',1),'TerminationMsg',struct('Selected','no','Byte0','0x00','Byte1','0x00','Byte2','0x00','Byte3','0x00','Byte4','0x00','Byte5','0x00','Byte6','0x00','Byte7','0x00'),'InitialMsg',struct('Selected','no','Byte0','0x00','Byte1','0x00','Byte2','0x00','Byte3','0x00','Byte4','0x00','Byte5','0x00','Byte6','0x00','Byte7','0x00'),'TriggerPort',struct('Selected','no','TriggerType','rising'),'BoardType','DS4302','BoardNo',1,'ControllerNo',1,'SFcnPortType','Scalar'),'TLCFileName','rtican_tx_message')
      settings: AttributesFormatString=Group Id: RTICAN1\n  SourceProductName=dSPACE RTI CAN Blockset
  wires:
  NERROW_LANE_SUPPORT_ST/1 -> Bus Selector1/1
  Bus Selector1/4 -> Data Type Conversion3/1  "<l_c1>"
  Bus Selector1/3 -> Data Type Conversion2/1  "<l_start_x0>"
  Bus Selector1/5 -> Data Type Conversion4/1  "<l_c2>"
  Bus Selector1/2 -> Data Type Conversion1/1  "<l_end_x0>"
  Bus Selector1/6 -> Data Type Conversion5/1  "<l_line_type>"
  Bus Selector1/1 -> Data Type Conversion/1  "<l_c0>"
  Bus Selector1/9 -> Data Type Conversion8/1  "<r_start_x0>"
  Bus Selector1/8 -> Data Type Conversion7/1  "<r_end_x0>"
  Bus Selector1/10 -> Data Type Conversion9/1  "<r_c1>"
  Bus Selector1/7 -> Data Type Conversion6/1  "<r_c0>"
  Bus Selector1/11 -> Data Type Conversion10/1  "<r_c2>"
  Bus Selector1/12 -> Data Type Conversion11/1  "<r_line_type>"
  Data Type Conversion/1 -> ZOP_NarrowLine_1/1
  Data Type Conversion1/1 -> ZOP_NarrowLine_1/2
  Data Type Conversion2/1 -> ZOP_NarrowLine_1/3
  Data Type Conversion3/1 -> ZOP_NarrowLine_1/4
  Data Type Conversion4/1 -> ZOP_NarrowLine_1/5
  Data Type Conversion5/1 -> ZOP_NarrowLine_1/6
  Data Type Conversion6/1 -> ZOP_NarrowLine_2/1
  Data Type Conversion7/1 -> ZOP_NarrowLine_2/2
  Data Type Conversion8/1 -> ZOP_NarrowLine_2/3
  Data Type Conversion9/1 -> ZOP_NarrowLine_2/4
  Data Type Conversion10/1 -> ZOP_NarrowLine_2/5
  Data Type Conversion11/1 -> ZOP_NarrowLine_2/6

== system LM_TOS_0107_FIX/LM_TOS_MODEL/adapter1 ==
  Fus_obj_outPut_st : Inport  OutDataTypeStr=Bus: FUS_OBJ_OUTPUT_ST
  Veh_State_st : Inport  Port=2  OutDataTypeStr=Bus: VSI_VEHSTATE_ST
  Fus_Lane_output_st : Inport  Port=3  OutDataTypeStr=Bus: FUS_LANE_OUTPUT_ST
  Fus_RoadEdge_output_st : Inport  Port=4  OutDataTypeStr=Bus: FUS_ROAD_EDGE_OUTPUT_ST
  acc_po_output_st : Inport  Port=5  OutDataTypeStr=Bus: ATS_PO_ST
  Bus Selector : BusSelector  OutputSignals=timeStamp,frameNum,objects
  Subsystem : Subsystem
  timeStamp : Outport
  frameNum : Outport  Port=2
  objects : Outport  Port=3
  veh_state : Outport  Port=4
  fus_lane_output : Outport  Port=5
  fus_RoadEdge_output : Outport  Port=6  OutDataTypeStr=Bus: FUS_ROAD_EDGE_OUTPUT_ST
  acc_po_st : Outport  Port=7  OutDataTypeStr=Bus: ATS_PO_ST
  wires:
  Fus_obj_outPut_st/1 -> Bus Selector/1
  Bus Selector/3 -> Subsystem/1(In3)  "<objects>"
  Bus Selector/1 -> timeStamp/1  "<timeStamp>"
  Bus Selector/2 -> frameNum/1  "<frameNum>"
  Subsystem/1(Out2) -> objects/1
  Veh_State_st/1 -> veh_state/1
  Fus_Lane_output_st/1 -> fus_lane_output/1
  Fus_RoadEdge_output_st/1 -> fus_RoadEdge_output/1
  acc_po_output_st/1 -> acc_po_st/1

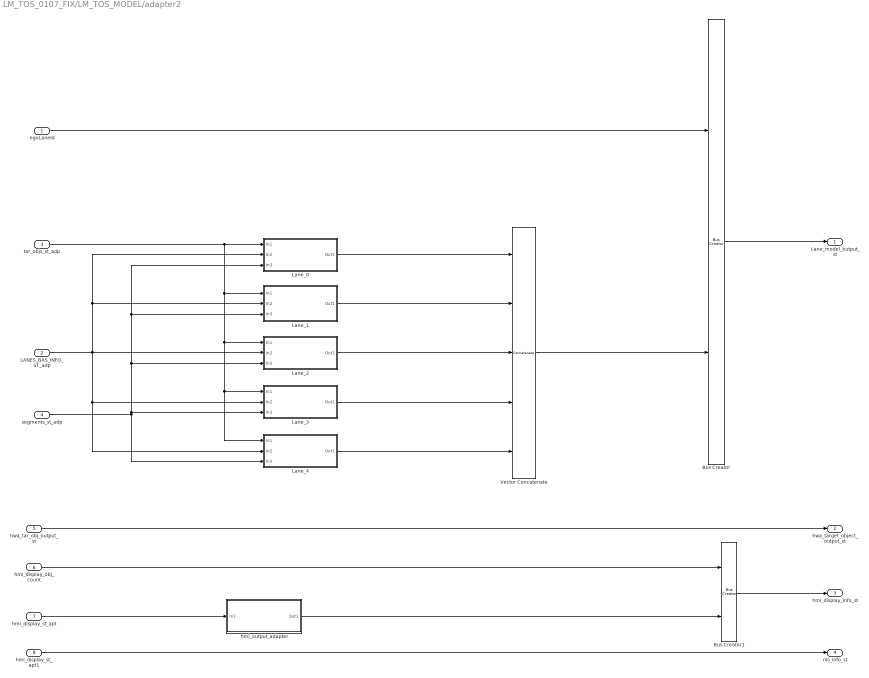
== system LM_TOS_0107_FIX/LM_TOS_MODEL/adapter2 ==
  egoLaneId : Inport  OutDataTypeStr=uint8
  LANES_BAS_INFO_ST_adp : Inport  Port=2  OutDataTypeStr=Bus: LANES_BAS_INFO_ST_adt
  tar_objs_st_adp : Inport  Port=3  OutDataTypeStr=Bus: TARGETOBJECTS_ST_adp
  segments_st_adp : Inport  Port=4  OutDataTypeStr=Bus: SEGMENTS_ST_adp
  hwa_tar_obj_output_st : Inport  Port=5  OutDataTypeStr=Bus: HWA_TARGETOBJECT_OUTPUT_ST
  hmi_display_obj_count : Inport  Port=6  OutDataTypeStr=uint8
  hmi_display_st_apt : Inport  Port=7  OutDataTypeStr=Bus: HMI_OUTPUT_ST_APT
  hmi_display_st_apt1 : Inport  Port=8  OutDataTypeStr=Bus: NARROW_LANE_SUPPORT_OUTPUT_ST
  Bus Creator : BusCreator  Inputs=2
  Bus Creator1 : BusCreator  Inputs=2
  Lane_0 : Subsystem
  Lane_1 : Subsystem
  Lane_2 : Subsystem
  Lane_3 : Subsystem
  Lane_4 : Subsystem
  Vector Concatenate : Concatenate  NumInputs=5
  hmi_output_adapter : Subsystem
  Lane_model_output_st : Outport  OutDataTypeStr=Bus: LANEMODEL_OUTPUT_ST
  hwa_target_object_output_st : Outport  Port=2  OutDataTypeStr=Bus: HWA_TARGETOBJECT_OUTPUT_ST
  hmi_display_info_st : Outport  Port=3  OutDataTypeStr=Bus: HMI_OUTPUT_ST
  nls_info_st : Outport  Port=4  OutDataTypeStr=Bus: NARROW_LANE_SUPPORT_OUTPUT_ST
  wires:
  hwa_tar_obj_output_st/1 -> hwa_target_object_output_st/1
  egoLaneId/1 -> Bus Creator/1
  tar_objs_st_adp/1 -> Lane_0/1(In1), Lane_2/1(In1), Lane_4/1(In1), Lane_3/1(In1), Lane_1/1(In1)
  LANES_BAS_INFO_ST_adp/1 -> Lane_4/2(In2), Lane_3/2(In2), Lane_2/2(In2), Lane_1/2(In2), Lane_0/2(In2)
  segments_st_adp/1 -> Lane_3/3(In3), Lane_2/3(In3), Lane_1/3(In3), Lane_0/3(In3), Lane_4/3(In3)
  Lane_1/1(Out1) -> Vector Concatenate/2
  Lane_2/1(Out1) -> Vector Concatenate/3
  Lane_0/1(Out1) -> Vector Concatenate/1
  Lane_3/1(Out1) -> Vector Concatenate/4
  Lane_4/1(Out1) -> Vector Concatenate/5
  Vector Concatenate/1 -> Bus Creator/2
  Bus Creator/1 -> Lane_model_output_st/1
  hmi_display_st_apt/1 -> hmi_output_adapter/1(In1)
  Bus Creator1/1 -> hmi_display_info_st/1
  hmi_display_obj_count/1 -> Bus Creator1/1
  hmi_output_adapter/1(Out1) -> Bus Creator1/2
  hmi_display_st_apt1/1 -> nls_info_st/1

== system LM_TOS_0107_FIX/RTI Data/RTI Data Store ==
  RTI Data Store : Subsystem  mask(RTI_DATA_STORE){}
      mask help:
      | RTI Data Store Block. This block is used by RTI to store internal model dependent data. Deleting this block will result in data loss.
      |
      | NEVER DELETE, COPY, OR MODIFY THIS BLOCK!
      mask Help:
      | RTI Data Store Block. This block is used by RTI to store internal model dependent data. Deleting this block will result in data loss.
      | 
      | NEVER DELETE, COPY, OR MODIFY THIS BLOCK!
      mask Display: text(0.5, 0.5, ' ', 'HorizontalAlignment', 'center');
